simulink model "planner_contral"  (R2023b)
settings: Solver=FixedStepAuto  StartTime=0  StopTime=inf  FixedStep=0.001  RelTol=1e-3
undefined symbols (not defined in the file): aubr, c_factor, cf, cr, iniObsHeading1, iniObsHeading2, iniObsPos1, iniObsPos2, KD_PID_distance, KD_PID_speed, KI_PID_distance, KI_PID_speed, KP_PID_distance, KP_PID_speed, la, lb, LQR_K1, LQR_K2, LQR_K3, LQR_K4, m, rack_displacement, refInfo_obs1, refInfo_obs2, right_wheel_ground, rightWaypoints, tablebr, vubr, vx_break_point
libraries: Solver_SF x1
(part 2 of 8)

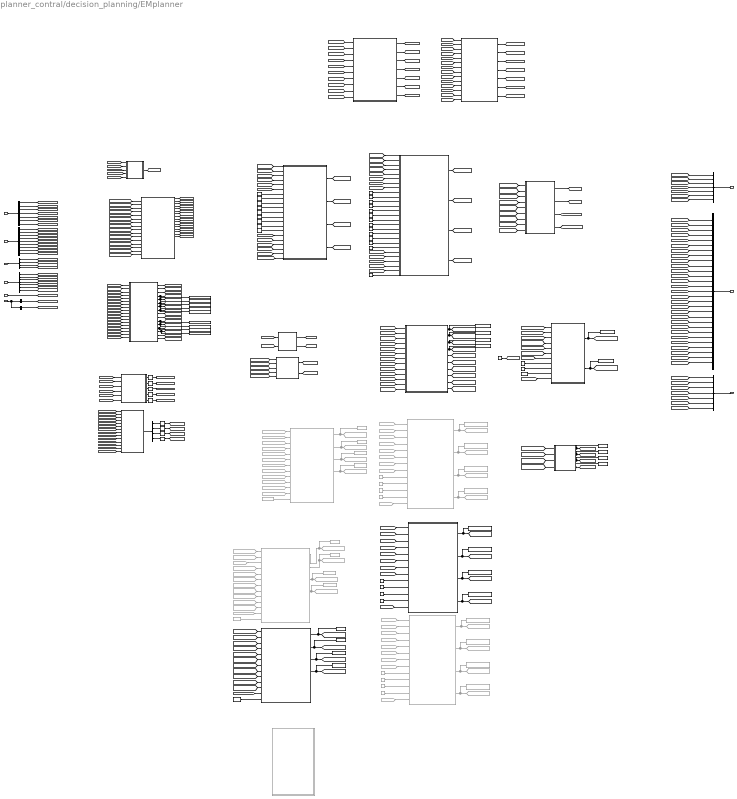
== system planner_contral/decision_planning/EMplanner ==
  note: 找到规划的起点
  note: 相对规划起点的时间序列
  note: 每个时刻对应的纵向位置
  note: 把QP的稀疏纵向轨迹增密、输出给后续控制器使用
  note: 在时域凸约束走廊内，对DP粗解进行平滑，求一条更连续、更舒适、更满足动力学约束的纵向轨迹。
  note: 路径速度拼接
  note: 在各个离散时刻上，静态/动态障碍物在ST图上占据的S下界和上界
  note: 输出
  note: 速度规划
  note: 路径索引到弧长的映射
  note: 当前规划起点处的纵向速度
  note: 当前规划起点横纵向位置
  note: 动态障碍物纵向速度
  note: 当前已生成的路径点，在 Frenet 下的轨迹
  note: 动态障碍物在 Frenet 下的位置和航向
  note: 静态障碍物在frenet下的位置和航向
  note: 把一条离散轨迹 (x,y) 转换成弧长坐标 s，并计算整条轨迹的总长度。
  note: 对给定的笛卡尔点，在参考线上搜索匹配点，并基于匹配点局部切线构造连续投影点，从而为后续 Frenet 坐标与动力学量转换提供基础几何信息。
  note: 点到参考线的匹配与投影函数
  note: 静态障碍物s
  note: 自车位置、航向角
  note: 上一周期轨迹 + 当前车辆状态
      | ↓
      | 判断是否还能沿用上一周期轨迹
      | ↓
      | 得到：
      | 1) 本周期规划起点
      | 2) 待拼接轨迹 stitch_trajectory
  note: 上一时刻规划的结果
      |
      | 当前时刻
      |
      | 自车信息
  note: 连续坐标：
      | s（沿道路方向）
      | l（横向偏移）
  note: origin = 自车在参考线上的投影点
  note: 这个模块的作用是：
      | 把参考线上的“点索引 i”转换成“弧长 s”，并且以自车投影点为 s=0
      | 构建以自车为原点的弧长坐标 s，实现“路径点编号 → 物理距离”的转换。。
  note: 输入
  note: 轨迹拼接计算模块
  note: accumulated_s计算模块
  note: 面向路径-速度解耦规划的障碍物预处理、参考线投影与动态轨迹构造模块
  note: 本周期规划起点
      |
      | 拼接轨迹
  note: （最多32）障碍物位置、速度、航向角
  note: 参考线位置、航向角、曲率
  note: 以自车为原点的弧长坐标 s
  note: 预测轨迹
  note: 静态障碍物l
  note: 静态障碍物航向角
  note: 动态障碍物s
  note: 动态障碍物l
  note: 动态障碍物s.
  note: 动态障碍物l.
  note: 动态障碍物航向角
  note: 本周期规划起点投影到参考线并转换到Frenet
  note: DP粗解决策+QP优化规划
      | 先离散决策，后连续优化。
  note: 每个时刻对应的纵向速度
  note: 每个时刻对应的纵向加速度
  note: 路径点的纵向坐标索引
  note: 当前规划时刻的绝对时间
  note: 把速度DP在ST图上的粗解转换成速度QP可直接使用的时域凸约束走廊。
  note: 路径规划
  referenceline_info : Inport
  location_info : Inport  Port=2
  perception info : Inport  Port=3
  pre_planning_info : Inport  Port=4
  current_time : Inport  Port=5
  visual_data : Inport  Port=6
  Bus Creator : BusCreator  Inputs=7
  Bus Creator1 : BusCreator  Inputs=29
  Bus Creator2 : BusCreator  Inputs=7
  Bus Selector : BusSelector  OutputSignals=smooth_ref_x,smooth_ref_y,smooth_ref_heading_,smooth_ref_kappa_,smooth_match_point_index,origin_x,origin_y
  Bus Selector1 : BusSelector  OutputSignals=ego_x,ego_y,ego_heading,ego_vx,ego_vy,ego_yaw_rate,ego_speed,ego_ax,ego_ay
  Bus Selector2 : BusSelector  OutputSignals=obs_x_set_gcs,obs_y_set_gcs,obs_velocity_set_gcs,obs_heading_set_gcs
  Bus Selector3 : BusSelector  OutputSignals=trajectory_x_gcs,trajectory_y_gcs,trajectory_heading_gcs,trajectory_kappa_gcs,trajectory_speed_gcs,trajectory_accel_gcs,trajectory_time_gcs
  Bus Selector4 : BusSelector  OutputSignals=preTraj_real1  OutputAsBus=on
  Bus Selector5 : BusSelector  OutputSignals=s_set,l_set,dl_set,ddl_set
  Bus Selector6 : BusSelector  OutputSignals=preTraj_real2  OutputAsBus=on
  Cartesian2Frenet : Subsystem
  Constant1 : Constant  Value=10
  Constant10 : Constant  Value=500
  Constant11 : Constant  Value=1000
  Constant12 : Constant  Value=500
  Constant13 : Constant  Value=100
  Constant{2,14,16,29} (4 alike) : Constant  Commented=on  Value=500
  Constant15 : Constant  Commented=on  Value=1000
  Constant17 : Constant  Commented=on  Value=100
  Constant18 : Constant  Commented=on  Value=0.2*9.8
  Constant28 : Constant  Commented=on  Value=1000
  Constant3 : Constant  Value=25
  Constant4 : Constant  Value=4000
  Constant5 : Constant  Value=100
  Constant6 : Constant  Value=1e8
  Constant60 : Constant  Value=1e8
  Constant61 : Constant  Value=1000
  Constant62 : Constant  Value=2
  Constant63 : Constant  Value=3
  Constant64 : Constant  Value=3
  Constant65 : Constant  Value=11
  Constant66 : Constant  Value=4
  Constant{67,76..78} (4 alike) : Constant  Value=15
  Constant68 : Constant  Value=1.2
  Constant69 : Constant  Value=0.1
  Constant7 : Constant  Commented=on  Value=0.2*9.8
  Constant70 : Constant  Value=0.02
  Constant71 : Constant  Value=2000
  Constant72 : Constant  Value=2500
  Constant73 : Constant  Value=50
  Constant74 : Constant  Value=20
  Constant75 : Constant  Value=5
  Constant79 : Constant  Value=2.5
  Constant8 : Constant  Value=0.2*9.8
  Constant80 : Constant  Value=2.5
  Constant81 : Constant  Value=1.6
  Constant9 : Constant  Commented=on  Value=100
  Frenet2Cartesian task : MATLAB Function  TreatAsAtomicUnit=on
  From{17,28,73,78} (4 alike) : From  Commented=on  GotoTag=obs_st_t_lb
  From{18,29,74,79} (4 alike) : From  Commented=on  GotoTag=obs_st_t_ub
  From{31,60,81,230} (4 alike) : From  Commented=on  GotoTag=dp_speed_s
  From231 : From  Commented=on  GotoTag=plan_start_s_dot
  From233 : From  Commented=on  GotoTag=plan_start_s_dot2
  From{32,63,82,234} (4 alike) : From  Commented=on  GotoTag=dp_speed_t
  From235 : From  Commented=on  GotoTag=s_lb
  From236 : From  Commented=on  GotoTag=s_ub
  From237 : From  Commented=on  GotoTag=s_dot_lb
  From238 : From  Commented=on  GotoTag=s_dot_ub
  From239 : From  Commented=on  GotoTag=reference_speed
  From25 : From  Commented=on  GotoTag=trajectory_kappa_init
  From26 : From  Commented=on  GotoTag=dynamic_s_lb
  From27 : From  Commented=on  GotoTag=dynaimc_s_ub
  From30 : From  Commented=on  GotoTag=path_s
  From33 : From  Commented=on  GotoTag=static_s_lb
  From34 : From  Commented=on  GotoTag=static_s_ub
  From61 : From  Commented=on  GotoTag=plan_start_s_dot
  From62 : From  Commented=on  GotoTag=plan_start_s_dot2
  From64 : From  Commented=on  GotoTag=s_lb
  From66 : From  Commented=on  GotoTag=s_ub
  From67 : From  Commented=on  GotoTag=s_dot_lb
  From71 : From  Commented=on  GotoTag=s_dot_ub
  From72 : From  Commented=on  GotoTag=reference_speed
  From75 : From  Commented=on  GotoTag=trajectory_kappa_init
  From76 : From  Commented=on  GotoTag=dynamic_s_lb
  From77 : From  Commented=on  GotoTag=dynaimc_s_ub
  From80 : From  Commented=on  GotoTag=path_s
  From83 : From  Commented=on  GotoTag=static_s_lb
  From84 : From  Commented=on  GotoTag=static_s_ub
  Goto146 : Goto  Commented=on  GotoTag=qp_s_init
  Goto147 : Goto  Commented=on  GotoTag=qp_s_dot_init
  Goto148 : Goto  Commented=on  GotoTag=qp_s_dot2_init
  Goto149 : Goto  Commented=on  GotoTag=relative_time_init
  Goto35 : Goto  Commented=on  GotoTag=s_lb
  Goto36 : Goto  Commented=on  GotoTag=s_ub
  Goto56 : Goto  Commented=on  GotoTag=s_dot_lb
  Goto57 : Goto  Commented=on  GotoTag=s_dot_ub
  Goto77 : Goto  Commented=on  GotoTag=qp_s_init
  Goto78 : Goto  Commented=on  GotoTag=qp_s_dot_init
  Goto79 : Goto  Commented=on  GotoTag=qp_s_dot2_init
  Goto80 : Goto  Commented=on  GotoTag=relative_time_init
  Goto81 : Goto  Commented=on  GotoTag=s_lb
  Goto82 : Goto  Commented=on  GotoTag=s_ub
  Goto83 : Goto  Commented=on  GotoTag=s_dot_lb
  Goto84 : Goto  Commented=on  GotoTag=s_dot_ub
  MATLAB Function1 : MATLAB Function  TreatAsAtomicUnit=on
  Selector{10..18} (9 alike) : Selector  InputPortWidth=128  IndexOptions=Index vector (dialog)  Indices=1  OutputSizes=1
  To Workspace : ToWorkspace  VariableName=log_dynamic_obs_s_set  SampleTime=-1
  To Workspace1 : ToWorkspace  VariableName=log_qp_s_init  SampleTime=-1
  To Workspace10 : ToWorkspace  VariableName=log_dp_speed_s  SampleTime=-1
  To Workspace11 : ToWorkspace  VariableName=log_dp_speed_t  SampleTime=-1
  To Workspace12 : ToWorkspace  Commented=on  VariableName=log_qp_s_init  SampleTime=-1
  To Workspace13 : ToWorkspace  Commented=on  VariableName=log_qp_s_dot_init  SampleTime=-1
  To Workspace14 : ToWorkspace  Commented=on  VariableName=log_qp_s_dot2_init  SampleTime=-1
  To Workspace15 : ToWorkspace  Commented=on  VariableName=log_relative_time_init  SampleTime=-1
  To Workspace16 : ToWorkspace  VariableName=log_s  SampleTime=-1
  To Workspace17 : ToWorkspace  VariableName=log_s_dot  SampleTime=-1
  To Workspace18 : ToWorkspace  VariableName=log_s_dot2  SampleTime=-1
  To Workspace19 : ToWorkspace  VariableName=log_relative_time  SampleTime=-1
  To Workspace2 : ToWorkspace  VariableName=log_static_s_lb  SampleTime=-1
  To Workspace20 : ToWorkspace  VariableName=log_dynamic_obs_l_set  SampleTime=-1
  To Workspace21 : ToWorkspace  VariableName=log_dynamic_obs_s_dot_set  SampleTime=-1
  To Workspace22 : ToWorkspace  VariableName=log_dynamic_obs_l_dot_set  SampleTime=-1
  To Workspace23 : ToWorkspace  VariableName=log_dynamic_obs_heading_set  SampleTime=-1
  To Workspace24 : ToWorkspace  VariableName=log_dynamic_obs_tra_x  SampleTime=-1
  To Workspace25 : ToWorkspace  VariableName=log_dynamic_obs_tra_y  SampleTime=-1
  To Workspace26 : ToWorkspace  VariableName=log_dynamic_obs_vx  SampleTime=-1
  To Workspace27 : ToWorkspace  VariableName=log_dynamic_obs_vy  SampleTime=-1
  To Workspace28 : ToWorkspace  Commented=on  VariableName=log_s_lb2  SampleTime=-1
  To Workspace29 : ToWorkspace  VariableName=log_s_lb  SampleTime=-1
  To Workspace3 : ToWorkspace  VariableName=log_static_s_ub  SampleTime=-1
  To Workspace30 : ToWorkspace  VariableName=log_s_ub  SampleTime=-1
  To Workspace31 : ToWorkspace  VariableName=log_s_dot_lb  SampleTime=-1
  To Workspace32 : ToWorkspace  VariableName=log_s_dot_ub  SampleTime=-1
  To Workspace33 : ToWorkspace  VariableName=log_qp_s_dot_init  SampleTime=-1
  To Workspace34 : ToWorkspace  VariableName=log_qp_s_dot2_init  SampleTime=-1
  To Workspace35 : ToWorkspace  VariableName=log_relative_time_init  SampleTime=-1
  To Workspace36 : ToWorkspace  Commented=on  VariableName=log_qp_s_init2  SampleTime=-1
  To Workspace37 : ToWorkspace  Commented=on  VariableName=log_qp_s_dot_init2  SampleTime=-1
  To Workspace38 : ToWorkspace  Commented=on  VariableName=log_qp_s_dot2_init2  SampleTime=-1
  To Workspace39 : ToWorkspace  Commented=on  VariableName=log_relative_time_init2  SampleTime=-1
  To Workspace4 : ToWorkspace  Commented=on  VariableName=log_s_lb  SampleTime=-1
  To Workspace40 : ToWorkspace  Commented=on  VariableName=log_s_ub2  SampleTime=-1
  To Workspace41 : ToWorkspace  Commented=on  VariableName=log_s_dot_lb2  SampleTime=-1
  To Workspace42 : ToWorkspace  Commented=on  VariableName=log_s_dot_ub2  SampleTime=-1
  To Workspace5 : ToWorkspace  Commented=on  VariableName=log_s_ub  SampleTime=-1
  To Workspace6 : ToWorkspace  Commented=on  VariableName=log_s_dot_lb  SampleTime=-1
  To Workspace7 : ToWorkspace  Commented=on  VariableName=log_s_dot_ub  SampleTime=-1
  To Workspace8 : ToWorkspace  VariableName=log_dynamic_s_lb  SampleTime=-1
  To Workspace9 : ToWorkspace  VariableName=log_dynamic_s_ub  SampleTime=-1
  calc path length and map between point and s : MATLAB Function  TreatAsAtomicUnit=on
  calc plan start info and stitch trajectory : MATLAB Function  TreatAsAtomicUnit=on
  calc speed planning start condition : MATLAB Function  TreatAsAtomicUnit=on
  generate convex space : MATLAB Function  Commented=on  TreatAsAtomicUnit=on
  generate convex space_base : MATLAB Function  TreatAsAtomicUnit=on
  generate convex space_new1 : MATLAB Function  Commented=on  TreatAsAtomicUnit=on
  generate st graph : MATLAB Function  TreatAsAtomicUnit=on
  generate st graph_base : MATLAB Function  Commented=on  TreatAsAtomicUnit=on
  genrate index to s : MATLAB Function  TreatAsAtomicUnit=on
  increase st point count : MATLAB Function  TreatAsAtomicUnit=on
  obs : Subsystem
  path and speed merge : MATLAB Function  TreatAsAtomicUnit=on
  path decision task : Subsystem
  path planning task : Subsystem
  spee planning with quadratic programming (qp) : MATLAB Function  Commented=on  TreatAsAtomicUnit=on
  spee planning with quadratic programming (qp)_1 : MATLAB Function  Commented=on  TreatAsAtomicUnit=on
  spee planning with quadratic programming (qp)_base : MATLAB Function  TreatAsAtomicUnit=on
  speed decision with dynamic planning(dp) : MATLAB Function  TreatAsAtomicUnit=on
  stitch trajectory : MATLAB Function  TreatAsAtomicUnit=on
  EM Planner result : Outport
  plot_visual : Outport  Port=2
  tra_ref_info : Outport  Port=3
  wires:
  referenceline_info/1 -> Bus Selector/1
  Bus Selector/1 -> [referenceline_x]  "<smooth_ref_x>"
  Bus Selector/2 -> [referenceline_y]  "<smooth_ref_y>"
  Bus Selector/3 -> [referenceline_heading]  "<smooth_ref_heading_>"
  Bus Selector/4 -> [referenceline_kappa]  "<smooth_ref_kappa_>"
  Bus Selector/5 -> [match_point_index]  "<smooth_match_point_index>"
  Bus Selector/6 -> [origin_x]  "<origin_x>"
  Bus Selector/7 -> [origin_y]  "<origin_y>"
  location_info/1 -> Bus Selector1/1
  Bus Selector1/1 -> [host_x]  "<ego_x>"
  Bus Selector1/2 -> [host_y]  "<ego_y>"
  Bus Selector1/3 -> [host_heading]  "<ego_heading>"
  Bus Selector1/4 -> [host_vx]  "<ego_vx>"
  Bus Selector1/5 -> [host_vy]  "<ego_vy>"
  Bus Selector1/6 -> [host_yawrate]  "<ego_yaw_rate>"
  Bus Selector1/7 -> [host_speed]  "<ego_speed>"
  Bus Selector1/8 -> [host_ax]  "<ego_ax>"
  Bus Selector1/9 -> [host_ay]  "<ego_ay>"
  pre_planning_info/1 -> Bus Selector3/1
  current_time/1 -> [current_time]
  [referenceline_y] -> genrate index to s/2(path_y)
  [referenceline_x] -> genrate index to s/1(path_x)
  genrate index to s/1(index2s) -> [index2s]
  [origin_y] -> genrate index to s/4(origin_y)
  [match_point_index] -> genrate index to s/5(origin_match_point_index)
  [origin_x] -> genrate index to s/3(origin_x)
  [host_ax] -> calc plan start info and stitch trajectory/14(host_ax)
  [host_ay] -> calc plan start info and stitch trajectory/15(host_ay)
  [pre_trajectory_x] -> calc plan start info and stitch trajectory/1(pre_trajectory_x)
  [pre_trajectory_y] -> calc plan start info and stitch trajectory/2(pre_trajectory_y)
  [pre_trajectory_heading] -> calc plan start info and stitch trajectory/3(pre_trajectory_heading)
  [pre_trajectory_kappa] -> calc plan start info and stitch trajectory/4(pre_trajectory_kappa)
  [pre_trajectory_speed] -> calc plan start info and stitch trajectory/5(pre_trajectory_velocity)
  [pre_trajectory_accel] -> calc plan start info and stitch trajectory/6(pre_trajectory_accel)
  [pre_trajectory_time] -> calc plan start info and stitch trajectory/7(pre_trajectory_time)
  [current_time] -> calc plan start info and stitch trajectory/8(current_time)
  [host_x] -> calc plan start info and stitch trajectory/9(host_x)
  [host_y] -> calc plan start info and stitch trajectory/10(host_y)
  [host_heading] -> calc plan start info and stitch trajectory/11(host_heading_xy)
  [host_vx] -> calc plan start info and stitch trajectory/12(host_vx)
  [host_vy] -> calc plan start info and stitch trajectory/13(host_vy)
  [host_speed] -> calc plan start info and stitch trajectory/16(host_speed)
  calc plan start info and stitch trajectory/1(plan_start_x) -> [plan_start_x_gcs]
  calc plan start info and stitch trajectory/2(plan_start_y) -> [plan_start_y_gcs]
  calc plan start info and stitch trajectory/4(plan_start_kappa) -> [plan_start_kappa_gcs]
  calc plan start info and stitch trajectory/5(plan_start_vx) -> [plan_start_vx_gcs]
  calc plan start info and stitch trajectory/6(plan_start_vy) -> [plan_start_vy_gcs]
  calc plan start info and stitch trajectory/7(plan_start_ax) -> [plan_start_ax_gcs]
  calc plan start info and stitch trajectory/8(plan_start_ay) -> [plan_start_ay_gcs]
  calc plan start info and stitch trajectory/9(plan_start_time) -> [plan_start_time]
  calc plan start info and stitch trajectory/11(stitch_y) -> [stitch_y_gcs]
  calc plan start info and stitch trajectory/12(stitch_heading) -> [stitch_heading_gcs]
  calc plan start info and stitch trajectory/13(stitch_kappa) -> [stitch_kappa_gcs]
  calc plan start info and stitch trajectory/14(stitch_speed) -> [stitch_speed_gcs]
  calc plan start info and stitch trajectory/15(stitch_accel) -> [stitch_accel_gcs]
  calc plan start info and stitch trajectory/16(stitch_time) -> [stitch_time]
  calc plan start info and stitch trajectory/3(plan_start_heading) -> [plan_start_heading_gcs]
  calc plan start info and stitch trajectory/10(stitch_x) -> [stitch_x_gcs]
  [plan_start_heading_gcs] -> calc speed planning start condition/5(plan_start_heading)
  [plan_start_ax_gcs] -> calc speed planning start condition/3(plan_start_ax)
  calc speed planning start condition/1(plan_start_s_dot) -> [plan_start_s_dot]
  [plan_start_vx_gcs] -> calc speed planning start condition/1(plan_start_vx)
  [plan_start_vy_gcs] -> calc speed planning start condition/2(plan_start_vy)
  [plan_start_ay_gcs] -> calc speed planning start condition/4(plan_start_ay)
  calc speed planning start condition/2(plan_start_s_dot2) -> [plan_start_s_dot2]
  calc path length and map between point and s/1(path_s_end) -> [path_s_end]
  calc path length and map between point and s/2(path_s) -> [path_s]  "path_s"
  [trajectory_x_init] -> calc path length and map between point and s/1(trajectory_x)
  [trajectory_y_init] -> calc path length and map between point and s/2(trajectory_y)
  Bus Creator/1 -> EM Planner result/1
  [trajectory_speed_final] -> Bus Creator/5  "trajectory_speed_gcs"
  [trajectory_time_final] -> Bus Creator/7  "trajectory_time_gcs"
  [trajectory_x_final] -> Bus Creator/1  "trajectory_x_gcs"
  [trajectory_kappa_final] -> Bus Creator/4  "trajectory_kappa_gcs"
  [trajectory_accel_final] -> Bus Creator/6  "trajectory_accel_gcs"
  [trajectory_heading_final] -> Bus Creator/3  "trajectory_heading_gcs"
  [trajectory_y_final] -> Bus Creator/2  "trajectory_y_gcs"
  Bus Selector3/1 -> [pre_trajectory_x]  "<trajectory_x_gcs>"
  Bus Selector3/7 -> [pre_trajectory_time]  "<trajectory_time_gcs>"
  Bus Selector3/6 -> [pre_trajectory_accel]  "<trajectory_accel_gcs>"
  Bus Selector3/5 -> [pre_trajectory_speed]  "<trajectory_speed_gcs>"
  Bus Selector3/4 -> [pre_trajectory_kappa]  "<trajectory_kappa_gcs>"
  Bus Selector3/3 -> [pre_trajectory_heading]  "<trajectory_heading_gcs>"
  Bus Selector3/2 -> [pre_trajectory_y]  "<trajectory_y_gcs>"
  [referenceline_x] -> obs/8(referenceline_x)
  [index2s] -> obs/12(index2s)
  [obs_velocity_set_gcs] -> obs/6(obs_velocity_set_gcs)
  [referenceline_heading] -> obs/10(referenceline_heading)
  [obs_heading_set_gcs] -> obs/7(obs_heading_set_gcs)
  [obs_x_set_gcs] -> obs/4(obs_x_set_gcs)
  [referenceline_kappa] -> obs/11(referenceline_kappa)
  [referenceline_y] -> obs/9(referenceline_y)
  obs/7(dynamic_obs_l_dot_set) -> [dynamic_obs_l_dot_set], To Workspace22/1
  [host_x] -> obs/1(host_x)
  obs/6(dynamic_obs_s_dot_set) -> [dynamic_obs_s_dot_set], To Workspace21/1
  obs/5(dynamic_obs_l_set) -> [dynamic_obs_l_set], To Workspace20/1
  [obs_y_set_gcs] -> obs/5(obs_y_set_gcs)
  obs/4(dynamic_obs_s_set) -> [dynamic_obs_s_set], To Workspace/1
  [host_heading] -> obs/3(host_heading_xy)
  [host_y] -> obs/2(host_y)
  Bus Selector2/4 -> [obs_heading_set_gcs]  "<obs_heading_set_gcs>"
  Bus Selector2/3 -> [obs_velocity_set_gcs]  "<obs_velocity_set_gcs>"
  Bus Selector2/1 -> [obs_x_set_gcs]  "<obs_x_set_gcs>"
  perception info/1 -> Bus Selector2/1
  Bus Selector2/2 -> [obs_y_set_gcs]  "<obs_y_set_gcs>"
  visual_data/1 -> Bus Selector6/1, Bus Selector4/1
  obs/1(static_obs_s_set) -> [static_obs_s_set]
  obs/2(static_obs_l_set) -> [static_obs_l_set]
  [path_s] -> obs/14(path_s)
  [preTraj1] -> obs/13(Pre_tra)
  [trajectory_x_init] -> obs/15(tra_x)
  [trajectory_y_init] -> obs/16(tra_y)
  [trajectory_kappa_init] -> obs/17(tra_kappa)
  [trajectory_heading_init] -> obs/18(tra_heaidng)
  obs/8(dynamic_obs_heading) -> [dynamic_obs_heading_set], To Workspace23/1
  obs/9(dynamic_obs_dl_set) -> [dynamic_obs_dl_set]
  obs/10(dynamic_obs_ddl_set) -> [dynamic_obs_ddl_set]
  obs/3(static_obs_heading_set) -> [static_obs_heading_set]
  obs/12(dynamic_obs_tra_y) -> [dynamic_obs_tra_y], To Workspace25/1
  obs/13(dynamic_obs_vx) -> To Workspace26/1, [dynamic_obs_vx]
  obs/14(dynamic_obs_vy) -> To Workspace27/1, [dynamic_obs_vy]
  obs/15(static_obs_x) -> [static_obs_x]
  obs/16(static_obs_y) -> [static_obs_y]
  obs/11(dynamic_obs_tra_x) -> [dynamic_obs_tra_x], To Workspace24/1
  [obs_st_t_ub] -> speed decision with dynamic planning(dp)/6(obs_st_t_ub)
  Constant6/1 -> speed decision with dynamic planning(dp)/10(w_cost_obs)
  [plan_start_s] -> generate st graph/12(plan_s)
  generate st graph/3(dynamic_obs_st_s_lb_set) -> To Workspace8/1, [dynamic_s_lb]
  generate st graph/7(static_obs_st_t_lb_set) -> [static_obs_st_t_in_set]
  [static_obs_l_set] -> generate st graph/2(static_obs_l)
  Constant5/1 -> speed decision with dynamic planning(dp)/9(w_cost_accel)
  speed decision with dynamic planning(dp)/2(dp_speed_t) -> To Workspace11/1, [dp_speed_t]
  generate st graph/2(static_obs_st_s_ub_set) -> To Workspace3/1, [static_s_ub]
  [obs_st_t_lb] -> speed decision with dynamic planning(dp)/5(obs_st_t_lb)
  [path_s] -> generate st graph/9(tra_path_indexs)
  generate st graph/1(static_obs_st_s_lb_set) -> To Workspace2/1, [static_s_lb]
  [qp_path_s_final] -> generate st graph/7(tra_s)
  Constant3/1 -> [reference_speed]
  [static_obs_s_set] -> generate st graph/1(static_obs_s)
  [plan_start_l] -> generate st graph/11(plan_l)
  [plan_start_s_dot] -> speed decision with dynamic planning(dp)/11(plan_start_s_dot)
  [dynaimc_s_ub] -> speed decision with dynamic planning(dp)/4(dynamic_obs_s_ub)
  speed decision with dynamic planning(dp)/1(dp_speed_s) -> To Workspace10/1, [dp_speed_s]
  [dynamic_s_lb] -> speed decision with dynamic planning(dp)/3(dynamic_obs_s_lb)
  [static_s_ub] -> speed decision with dynamic planning(dp)/2(static_obs_s_ub)
  Constant4/1 -> speed decision with dynamic planning(dp)/8(w_cost_ref_speed)
  [reference_speed] -> speed decision with dynamic planning(dp)/7(reference_speed_unlimit)
  [qp_path_l_final] -> generate st graph/8(tra_l)
  [static_obs_heading_set] -> generate st graph/3(static_obs_heading)
  [static_s_lb] -> speed decision with dynamic planning(dp)/1(static_obs_s_lb)
  [dynamic_obs_heading_set] -> generate st graph/6(dynamic_obs_heaidng_set)
  [dynamic_obs_l_set] -> generate st graph/5(dynamic_obs_l_set)
  [plan_start_s_dot] -> generate st graph/10(plan_s_dot)
  generate st graph/8(static_obs_st_t_ub_set) -> [static_obs_st_t_out_set]
  [dynamic_obs_s_dot_set] -> generate st graph/13(dynamic_obs_s_dot)
  generate st graph/4(dynamic_obs_st_s_ub_set) -> To Workspace9/1, [dynaimc_s_ub]
  [dynamic_obs_s_set] -> generate st graph/4(dynamic_obs_s_set)
  generate st graph/9(dynamic_obs_st_t_lb_set) -> [dynamic_obs_st_t_in_set]
  generate st graph/10(dynamic_obs_st_t_ub_set) -> [dynamic_obs_st_t_out_set]
  generate st graph/5(obs_st_t_lb_set) -> [obs_st_t_lb]
  generate st graph/6(obs_st_t_ub_set) -> [obs_st_t_ub]
  From236/1 -> spee planning with quadratic programming (qp)/6(s_ub)
  From230/1 -> spee planning with quadratic programming (qp)/3(dp_speed_s)
  From235/1 -> spee planning with quadratic programming (qp)/5(s_lb)
  From234/1 -> spee planning with quadratic programming (qp)/4(dp_speed_t)
  spee planning with quadratic programming (qp)/4(relative_time_init) -> To Workspace15/1, Goto149/1
  From239/1 -> spee planning with quadratic programming (qp)/13(speed_reference)
  From233/1 -> spee planning with quadratic programming (qp)/2(plan_start_s_dot2)
  From238/1 -> spee planning with quadratic programming (qp)/8(s_dot_ub)
  spee planning with quadratic programming (qp)/1(qp_s_init) -> To Workspace12/1, Goto146/1
  From237/1 -> spee planning with quadratic programming (qp)/7(s_dot_lb)
  From231/1 -> spee planning with quadratic programming (qp)/1(plan_start_s_dot)
  Constant9/1 -> spee planning with quadratic programming (qp)/9(w_cost_s_dot2)
  Constant29/1 -> spee planning with quadratic programming (qp)/11(w_cost_jerk)
  spee planning with quadratic programming (qp)/2(qp_s_dot_init) -> To Workspace13/1, Goto147/1
  spee planning with quadratic programming (qp)/3(qp_s_dot2_init) -> To Workspace14/1, Goto148/1
  Constant28/1 -> spee planning with quadratic programming (qp)/10(w_cost_v_ref)
  Constant2/1 -> spee planning with quadratic programming (qp)/12(w_ref_s)
  stitch trajectory/3(trajectory_heading_final) -> [trajectory_heading_final]
  [trajectory_x_init] -> path and speed merge/7(trajectory_x_init)
  [trajectory_kappa] -> stitch trajectory/4(trajectory_kappa)
  [trajectory_accel] -> stitch trajectory/6(trajectory_accel)
  [stitch_y_gcs] -> stitch trajectory/9(stitch_y)
  stitch trajectory/1(trajectory_x_final) -> [trajectory_x_final]
  stitch trajectory/2(trajectory_y_final) -> [trajectory_y_final]
  stitch trajectory/7(trajectory_time_final) -> [trajectory_time_final]
  [stitch_x_gcs] -> stitch trajectory/8(stitch_x)
  path and speed merge/4(trajectory_kappa) -> [trajectory_kappa]
  [trajectory_x] -> stitch trajectory/1(trajectory_x)
  stitch trajectory/4(trajectory_kappa_final) -> [trajectory_kappa_final]
  [relative_time] -> path and speed merge/4(relative_time)
  [s_dot2] -> path and speed merge/3(s_dot2)
  [plan_start_time] -> path and speed merge/5(current_time)
  increase st point count/3(s_dot2) -> To Workspace18/1, [s_dot2]
  [stitch_heading_gcs] -> stitch trajectory/10(stitch_heading)
  [trajectory_y] -> stitch trajectory/2(trajectory_y)
  increase st point count/2(s_dot) -> To Workspace17/1, [s_dot]
  [trajectory_y_init] -> path and speed merge/8(trajectory_y_init)
  stitch trajectory/5(trajectory_speed_final) -> [trajectory_speed_final]
  [trajectory_time] -> stitch trajectory/7(trajectory_time)
  [path_s] -> path and speed merge/6(path_s)
  [trajectory_heading_init] -> path and speed merge/9(trajectory_heading_init)
  path and speed merge/2(trajectory_y) -> [trajectory_y]
  [trajectory_heading] -> stitch trajectory/3(trajectory_heading)
  [stitch_kappa_gcs] -> stitch trajectory/11(stitch_kappa)
  path and speed merge/5(trajectory_speed) -> [trajectory_speed]
  path and speed merge/3(trajectory_heading) -> [trajectory_heading]
  [stitch_accel_gcs] -> stitch trajectory/13(stitch_accel)
  [stitch_speed_gcs] -> stitch trajectory/12(stitch_speed)
  [trajectory_speed] -> stitch trajectory/5(trajectory_speed)
  [s] -> path and speed merge/1(s)
  path and speed merge/7(trajectory_time) -> [trajectory_time]
  path and speed merge/6(trajectory_accel) -> [trajectory_accel]
  [qp_s_dot2_init] -> increase st point count/3(s_dot2_init)
  [relative_time_init] -> increase st point count/4(relative_time_init)
  [trajectory_kappa_init] -> path and speed merge/10(trajectory_kappa_init)
  [stitch_time] -> stitch trajectory/14(stitch_time)
  [qp_s_init] -> increase st point count/1(s_init)
  increase st point count/1(s) -> To Workspace16/1, [s]
  path and speed merge/1(trajectory_x) -> [trajectory_x]
  [s_dot] -> path and speed merge/2(s_dot)
  [qp_s_dot_init] -> increase st point count/2(s_dot_init)
  stitch trajectory/6(trajectory_accel_final) -> [trajectory_accel_final]
  increase st point count/4(relative_time) -> To Workspace19/1, [relative_time]
  [dynaimc_s_ub] -> Bus Creator1/17  "dynaimc_s_ub"
  [dynamic_s_lb] -> Bus Creator1/16  "dynamic_s_lb"
  [dp_path_s_final_ceshi] -> Bus Creator1/1  "dp_path_s_final_ceshi"
  [dp_path_l_final_ceshi] -> Bus Creator1/2  "dp_path_l_final_ceshi"
  [qp_path_s_final] -> Bus Creator1/3  "qp_path_s_final"
  [qp_path_l_final] -> Bus Creator1/4  "qp_path_l_final"
  [l_min] -> Bus Creator1/5  "l_min"
  [l_max] -> Bus Creator1/6  "l_max"
  [static_obs_s_set] -> Bus Creator1/7  "static_obs_s_set"
  [static_obs_l_set] -> Bus Creator1/8  "static_obs_l_set"
  [plan_start_s] -> Bus Creator1/9  "plan_start_s"
  [plan_start_l] -> Bus Creator1/10  "plan_start_l"
  [plan_start_dl] -> Bus Creator1/11  "plan_start_dl"
  [dynamic_obs_s_set] -> Bus Creator1/12  "dynamic_obs_s_set"
  [dynamic_obs_l_set] -> Bus Creator1/13  "dynamic_obs_l_set"
  [static_s_lb] -> Bus Creator1/14  "static_s_lb"
  [static_s_ub] -> Bus Creator1/15  "static_s_ub"
  [dp_speed_s] -> Bus Creator1/18  "dp_speed_s"
  [dp_speed_t] -> Bus Creator1/19  "dp_speed_t"
  [qp_s_init] -> Bus Creator1/20  "qp_s_init"
  [relative_time_init] -> Bus Creator1/21  "relative_time_init"
  [obs_st_t_lb] -> Bus Creator1/22  "obs_st_t_lb"
  [obs_st_t_ub] -> Bus Creator1/23  "obs_st_t_ub"
  [static_obs_st_t_in_set] -> Bus Creator1/24  "static_obs_st_t_in_set"
  [static_obs_st_t_out_set] -> Bus Creator1/25  "static_obs_st_t_out_set"
  [dynamic_obs_st_t_in_set] -> Bus Creator1/26  "dynamic_obs_st_t_in_set"
  [dynamic_obs_st_t_out_set] -> Bus Creator1/27  "dynamic_obs_st_t_out_set"
  [s_lb] -> Bus Creator1/28  "s_lb"
  [s_ub] -> Bus Creator1/29  "s_ub"
  Bus Creator1/1 -> plot_visual/1
  [referenceline_x] -> Bus Creator2/3  "referenceline_x"
  [trajectory_x_final] -> Bus Creator2/5  "trajectory_x_final"
  [host_y] -> Bus Creator2/2  "host_y"
  [referenceline_y] -> Bus Creator2/4  "referenceline_y"
  [trajectory_y_final] -> Bus Creator2/6  "trajectory_y_final"
  [host_x] -> Bus Creator2/1  "host_x"
  Bus Creator2/1 -> tra_ref_info/1
  [host_heading] -> Bus Creator2/7  "host_heading"
  path planning task/1(qp_path_s_final) -> [qp_path_s_final]
  Constant79/1 -> path planning task/17(host_d1)
  MATLAB Function1/4(proj_heading_set) -> Selector13/1
  [qp_path_s_final] -> Frenet2Cartesian task/1(s_set)
  [qp_path_dl_final] -> Frenet2Cartesian task/3(dl_set)
  [referenceline_heading] -> MATLAB Function1/5(frenet_path_heading)
  Frenet2Cartesian task/1(x_set) -> [trajectory_x_init]
  [referenceline_y] -> MATLAB Function1/4(frenet_path_y)
  [plan_start_match_point_index] -> Cartesian2Frenet/9(proj_match_point_index_set)
  [plan_start_vy_gcs] -> Cartesian2Frenet/4(vy_set)
  Selector11/1 -> [plan_start_proj_x]
  [referenceline_y] -> Cartesian2Frenet/8(frenet_path_y)
  [referenceline_x] -> Frenet2Cartesian task/5(frenet_path_x)
  [referenceline_kappa] -> Frenet2Cartesian task/8(frenet_path_kappa)
  Frenet2Cartesian task/2(y_set) -> [trajectory_y_init]
  MATLAB Function1/5(proj_kappa_set) -> Selector14/1
  [referenceline_x] -> Cartesian2Frenet/7(frenet_path_x)
  Bus Selector5/4 -> Selector18/1  "<ddl_set>"
  [plan_start_x_gcs] -> MATLAB Function1/1(x_set)
  Frenet2Cartesian task/4(kappa_set) -> [trajectory_kappa_init]
  [index2s] -> Frenet2Cartesian task/9(index2s)
  Bus Selector5/2 -> Selector16/1  "<l_set>"
  [plan_start_ax_gcs] -> Cartesian2Frenet/5(ax_set)
  [plan_start_vx_gcs] -> Cartesian2Frenet/3(vx_set)
  Selector15/1 -> [plan_start_s]
  Selector14/1 -> [plan_start_proj_kappa]
  Selector16/1 -> [plan_start_l]
  [plan_start_ay_gcs] -> Cartesian2Frenet/6(ay_set)
  [plan_start_proj_y] -> Cartesian2Frenet/11(proj_y_set)
  Selector17/1 -> [plan_start_dl]
  [index2s] -> Cartesian2Frenet/14(index2s)
  [referenceline_y] -> Frenet2Cartesian task/6(frenet_path_y)
  [dynamic_obs_s_dot_set] -> path decision task/18(dynamic_s_dot)
  MATLAB Function1/1(match_point_index_set) -> Selector10/1
  MATLAB Function1/2(proj_x_set) -> Selector11/1
  path decision task/1(dp_path_s_final) -> [dp_path_s_final_ceshi]
  [qp_path_ddl_final] -> Frenet2Cartesian task/4(ddl_set)
  Bus Selector5/1 -> Selector15/1  "<s_set>"
  [plan_start_s] -> path planning task/5(plan_start_s)
  Selector18/1 -> [plan_start_ddl]
  Constant64/1 -> path decision task/11(dp_cost_ref)
  [plan_start_s] -> path decision task/3(plan_start_s)
  Constant76/1 -> path planning task/14(qp_cost_endl)
  [referenceline_kappa] -> MATLAB Function1/6(frenet_path_kappa)
  Bus Selector5/3 -> Selector17/1  "<dl_set>"
  Constant74/1 -> path planning task/12(qp_cost_dddl)
  [plan_start_dl] -> path decision task/5(plan_start_dl)
  Constant66/1 -> path decision task/13(dp_col)
  [plan_start_proj_kappa] -> Cartesian2Frenet/13(proj_kappa_set)
  [dynamic_obs_l_dot_set] -> path decision task/19(dynamic_l_dot)
  Constant62/1 -> path decision task/9(dp_cost_ddl)
  path planning task/2(qp_path_l_final) -> [qp_path_l_final]
  path decision task/3(dp_path_dl_final) -> [dp_path_dl_final_ceshi]
  Constant81/1 -> path planning task/19(host_w)
  [dynamic_obs_s_set] -> path decision task/16(dynamic_s)
  Constant68/1 -> path decision task/15(dp_sample_l)
  [static_obs_s_set] -> path decision task/1(static_obs_s_set)
  Constant67/1 -> path decision task/14(dp_sample_s)
  path planning task/4(qp_path_ddl_final) -> [qp_path_ddl_final]
  [static_obs_l_set] -> path planning task/4(static_obs_l_set)
  [dynamic_obs_l_set] -> path decision task/17(dynamic_l)
  Constant71/1 -> path planning task/9(qp_cost_l)
  [static_obs_s_set] -> path planning task/3(static_obs_s_set)
  [dp_path_s_final_ceshi] -> path planning task/1(dp_path_s_final)
  Constant78/1 -> path planning task/16(qp_cost_end_ddl)
  Constant69/1 -> path planning task/20(delta_dl_max)
  [plan_start_ddl] -> path planning task/8(plan_start_ddl)
  path decision task/2(dp_path_l_final) -> [dp_path_l_final_ceshi]
  [referenceline_heading] -> Frenet2Cartesian task/7(frenet_path_heading)
  Constant73/1 -> path planning task/11(qp_cost_ddl)
  [plan_start_dl] -> path planning task/7(plan_start_dl)
  MATLAB Function1/3(proj_y_set) -> Selector12/1
  Cartesian2Frenet/1(Cartesian2FrenetOut) -> Bus Selector5/1
  [dynamic_obs_s_set] -> path planning task/22(dynamic_s)
  Constant70/1 -> path planning task/21(delta_ddl_max)
  [dynamic_obs_heading_set] -> path planning task/26(dynamic_heading)
  [dynamic_obs_l_set] -> path planning task/23(dynamic_l)
  Selector13/1 -> [plan_start_proj_heading]
  [dp_path_l_final_ceshi] -> path planning task/2(dp_path_l_final)
  Constant60/1 -> path decision task/7(dp_cost_collision)
  Constant63/1 -> path decision task/10(dp_cost_dddl)
  path planning task/3(qp_path_dl_final) -> [qp_path_dl_final]
  [qp_path_l_final] -> Frenet2Cartesian task/2(l_set)
  [static_obs_l_set] -> path decision task/2(static_obs_l_set)
  [referenceline_x] -> MATLAB Function1/3(frenet_path_x)
  [plan_start_l] -> path decision task/4(plan_start_l)
  Constant77/1 -> path planning task/15(qp_cost_end_dl)
  [dynamic_obs_l_dot_set] -> path planning task/25(dynamic_l_dot)
  Selector10/1 -> [plan_start_match_point_index]
  Selector12/1 -> [plan_start_proj_y]
  [dynamic_obs_s_dot_set] -> path planning task/24(dynamic_s_dot)
  [plan_start_ddl] -> path decision task/6(plan_start_ddl)
  Frenet2Cartesian task/3(heading_set) -> [trajectory_heading_init]
  [plan_start_l] -> path planning task/6(plan_start_l)
  [plan_start_proj_heading] -> Cartesian2Frenet/12(proj_heading_set)
  path decision task/4(dp_path_ddl_final) -> [dp_path_ddl_final_ceshi]
  [dynamic_obs_heading_set] -> path decision task/21(dynamic_obs_heading)
  [plan_start_proj_x] -> Cartesian2Frenet/10(proj_x_set)
  Constant72/1 -> path planning task/10(qp_cost_dl)
  [plan_start_x_gcs] -> Cartesian2Frenet/1(x_set)
  [plan_start_y_gcs] -> MATLAB Function1/2(y_set)
  Constant1/1 -> path planning task/27(w_ref_dp)
  [static_obs_heading_set] -> path decision task/20(static_obs_heading)
  Constant65/1 -> path decision task/12(dp_row)
  [plan_start_y_gcs] -> Cartesian2Frenet/2(y_set)
  Constant80/1 -> path planning task/18(host_d2)
  Constant75/1 -> path planning task/13(qp_cost_centre)
  Constant61/1 -> path decision task/8(dp_cost_dl)
  From33/1 -> generate convex space/4(static_obs_s_lb)
  From31/1 -> generate convex space/1(dp_speed_s)
  From27/1 -> generate convex space/9(dynamic_obs_s_ub)
  From26/1 -> generate convex space/8(dynamic_obs_s_lb)
  From29/1 -> generate convex space/11(dynamic_obs_t_ub)
  From28/1 -> generate convex space/10(dynamic_obs_t_lb)
  From32/1 -> generate convex space/2(dp_speed_t)
  From34/1 -> generate convex space/5(static_obs_s_ub)
  From17/1 -> generate convex space/6(static_obs_t_lb)
  From30/1 -> generate convex space/3(path_index2s)
  From18/1 -> generate convex space/7(static_obs_t_ub)
  generate convex space/1(s_lb) -> Goto35/1, To Workspace4/1
  From25/1 -> generate convex space/12(trajectory_kappa_init)
  Constant7/1 -> generate convex space/13(max_lateral_accel)
  generate convex space/2(s_ub) -> Goto36/1, To Workspace5/1
  generate convex space/4(s_dot_ub) -> Goto57/1, To Workspace7/1
  generate convex space/3(s_dot_lb) -> Goto56/1, To Workspace6/1
  Bus Selector4/1 -> [preTraj1]
  Bus Selector6/1 -> [preTraj2]
  Constant8/1 -> generate convex space_base/13(max_lateral_accel)
  [trajectory_kappa_init] -> generate convex space_base/12(trajectory_kappa_init)
  [obs_st_t_ub] -> generate convex space_base/7(static_obs_t_ub)
  [path_s] -> generate convex space_base/3(path_index2s)
  [obs_st_t_lb] -> generate convex space_base/6(static_obs_t_lb)
  [static_s_ub] -> generate convex space_base/5(static_obs_s_ub)
  [dp_speed_t] -> generate convex space_base/2(dp_speed_t)
  [obs_st_t_lb] -> generate convex space_base/10(dynaimc_obs_t_lb)
  [obs_st_t_ub] -> generate convex space_base/11(dynaimc_obs_t_ub)
  [dynamic_s_lb] -> generate convex space_base/8(dynamic_obs_s_lb)
  [dynaimc_s_ub] -> generate convex space_base/9(dynamic_obs_s_ub)
  [dp_speed_s] -> generate convex space_base/1(dp_speed_s)
  [static_s_lb] -> generate convex space_base/4(static_obs_s_lb)
  generate convex space_base/3(s_dot_lb) -> To Workspace31/1, [s_dot_lb]
  generate convex space_base/4(s_dot_ub) -> To Workspace32/1, [s_dot_ub]
  generate convex space_base/2(s_ub) -> To Workspace30/1, [s_ub]
  generate convex space_base/1(s_lb) -> To Workspace29/1, [s_lb]
  spee planning with quadratic programming (qp)_base/3(qp_s_dot2_init) -> [qp_s_dot2_init], To Workspace34/1
  spee planning with quadratic programming (qp)_base/2(qp_s_dot_init) -> [qp_s_dot_init], To Workspace33/1
  spee planning with quadratic programming (qp)_base/1(qp_s_init) -> [qp_s_init], To Workspace1/1
  spee planning with quadratic programming (qp)_base/4(relative_time_init) -> [relative_time_init], To Workspace35/1
  Constant10/1 -> spee planning with quadratic programming (qp)_base/12(w_ref_s)
  Constant11/1 -> spee planning with quadratic programming (qp)_base/10(w_cost_v_ref)
  Constant12/1 -> spee planning with quadratic programming (qp)_base/11(w_cost_jerk)
  Constant13/1 -> spee planning with quadratic programming (qp)_base/9(w_cost_s_dot2)
  [plan_start_s_dot] -> spee planning with quadratic programming (qp)_base/1(plan_start_s_dot)
  [s_dot_lb] -> spee planning with quadratic programming (qp)_base/7(s_dot_lb)
  [s_dot_ub] -> spee planning with quadratic programming (qp)_base/8(s_dot_ub)
  [plan_start_s_dot2] -> spee planning with quadratic programming (qp)_base/2(plan_start_s_dot2)
  [reference_speed] -> spee planning with quadratic programming (qp)_base/13(speed_reference)
  [dp_speed_t] -> spee planning with quadratic programming (qp)_base/4(dp_speed_t)
  [s_lb] -> spee planning with quadratic programming (qp)_base/5(s_lb)
  [dp_speed_s] -> spee planning with quadratic programming (qp)_base/3(dp_speed_s)
  [s_ub] -> spee planning with quadratic programming (qp)_base/6(s_ub)
  Constant14/1 -> spee planning with quadratic programming (qp)_1/12(w_ref_s)
  Constant15/1 -> spee planning with quadratic programming (qp)_1/10(w_cost_v_ref)
  spee planning with quadratic programming (qp)_1/3(qp_s_dot2_init) -> Goto79/1, To Workspace38/1
  spee planning with quadratic programming (qp)_1/2(qp_s_dot_init) -> Goto78/1, To Workspace37/1
  Constant16/1 -> spee planning with quadratic programming (qp)_1/11(w_cost_jerk)
  Constant17/1 -> spee planning with quadratic programming (qp)_1/9(w_cost_s_dot2)
  From61/1 -> spee planning with quadratic programming (qp)_1/1(plan_start_s_dot)
  From67/1 -> spee planning with quadratic programming (qp)_1/7(s_dot_lb)
  spee planning with quadratic programming (qp)_1/1(qp_s_init) -> Goto77/1, To Workspace36/1
  From71/1 -> spee planning with quadratic programming (qp)_1/8(s_dot_ub)
  From62/1 -> spee planning with quadratic programming (qp)_1/2(plan_start_s_dot2)
  From72/1 -> spee planning with quadratic programming (qp)_1/13(speed_reference)
  spee planning with quadratic programming (qp)_1/4(relative_time_init) -> Goto80/1, To Workspace39/1
  From63/1 -> spee planning with quadratic programming (qp)_1/4(dp_speed_t)
  From64/1 -> spee planning with quadratic programming (qp)_1/5(s_lb)
  From60/1 -> spee planning with quadratic programming (qp)_1/3(dp_speed_s)
  From66/1 -> spee planning with quadratic programming (qp)_1/6(s_ub)
  generate convex space_new1/1(s_lb) -> Goto81/1, To Workspace28/1
  generate convex space_new1/2(s_ub) -> Goto82/1, To Workspace40/1
  generate convex space_new1/4(s_dot_ub) -> Goto84/1, To Workspace42/1
  generate convex space_new1/3(s_dot_lb) -> Goto83/1, To Workspace41/1
  From83/1 -> generate convex space_new1/4(static_obs_s_lb)
  From81/1 -> generate convex space_new1/1(dp_speed_s)
  From77/1 -> generate convex space_new1/9(dynamic_obs_s_ub)
  From76/1 -> generate convex space_new1/8(dynamic_obs_s_lb)
  From79/1 -> generate convex space_new1/11(dynamic_obs_t_ub)
  From78/1 -> generate convex space_new1/10(dynamic_obs_t_lb)
  From82/1 -> generate convex space_new1/2(dp_speed_t)
  From84/1 -> generate convex space_new1/5(static_obs_s_ub)
  From73/1 -> generate convex space_new1/6(static_obs_t_lb)
  From80/1 -> generate convex space_new1/3(path_index2s)
  From74/1 -> generate convex space_new1/7(static_obs_t_ub)
  From75/1 -> generate convex space_new1/12(trajectory_kappa_init)
  Constant18/1 -> generate convex space_new1/13(max_lateral_accel)

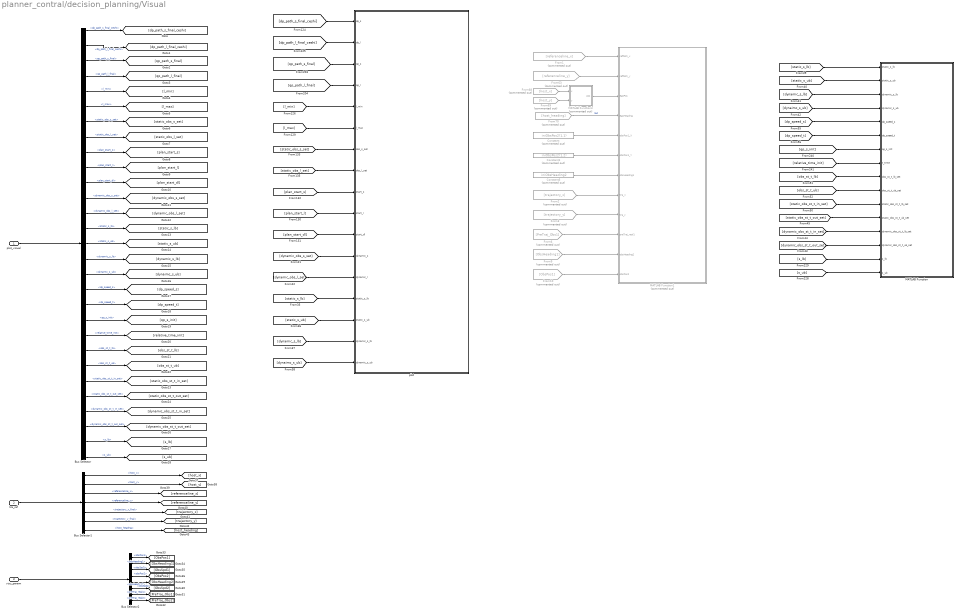
== system planner_contral/decision_planning/Visual ==
  plot_visual : Inport
  tra_ref : Inport  Port=2
  visu_param : Inport  Port=3
  Bus Selector : BusSelector  OutputSignals=dp_path_s_final_ceshi,dp_path_l_final_ceshi,qp_path_s_final,qp_path_l_final,l_min,l_max,static_obs_s_set,static_obs_l_set,plan_start_s,plan_start_l,plan_start_dl,dynamic_obs_s_set,dynamic_obs_l_set,static_s_lb,static_s_ub,dynamic_s_lb,dynaimc_s_ub,dp_speed_s,dp_speed_t,qp_s_init,relative_time_init,obs_st_t_lb,obs_st_t_ub,static_obs_st_t_in_set,static_obs_st_t_out_set,dynamic_obs_st_t_in_set,dynamic_obs_st_t_out_set,s_lb,s_ub
  Bus Selector1 : BusSelector  OutputSignals=host_x,host_y,referenceline_x,referenceline_y,trajectory_x_final,trajectory_y_final,host_heading
  Bus Selector2 : BusSelector  OutputSignals=obsPos1,obsHeading1,obsSpd1,obsPos2,obsHeading2,obsSpd2,preTraj_real1,preTraj_real2
  Constant : Constant  Commented=on  Value=iniObsPos2(1,1)
  Constant1 : Constant  Commented=on  Value=iniObsPos2(1,2)
  Constant5 : Constant  Commented=on  Value=iniObsHeading2
  From1 : From  Commented=on  GotoTag=referenceline_x
  From10 : From  Commented=on  GotoTag=ObsPos1
  From2 : From  Commented=on  GotoTag=trajectory_x
  From3 : From  Commented=on  GotoTag=trajectory_y
  From6 : From  Commented=on  GotoTag=PreTraj_Obs1
  From63 : From  Commented=on  GotoTag=referenceline_y
  From68 : From  Commented=on  GotoTag=host_x
  From69 : From  Commented=on  GotoTag=host_y
  From70 : From  Commented=on  GotoTag=host_heading
  From9 : From  Commented=on  GotoTag=ObsHeading1
  MATLAB Function : MATLAB Function  TreatAsAtomicUnit=on
  MATLAB Function1 : MATLAB Function  Commented=on  TreatAsAtomicUnit=on
  MATLAB Function3 : MATLAB Function  Commented=on  TreatAsAtomicUnit=on
  plot : MATLAB Function  TreatAsAtomicUnit=on
  wires:
  [qp_s_init] -> MATLAB Function/7(qp_s_init)
  [dp_speed_s] -> MATLAB Function/5(dp_speed_s)
  [dp_speed_t] -> MATLAB Function/6(dp_speed_t)
  [dynamic_obs_l_set] -> plot/13(dynamic_l)
  [qp_path_l_final] -> plot/4(qp_l)
  [s_ub] -> MATLAB Function/16(s_ub)
  [dp_path_l_final_ceshi] -> plot/2(dp_l)
  [static_obs_st_t_in_set] -> MATLAB Function/11(static_obs_st_t_lb_set)
  [static_s_ub] -> plot/15(static_s_ub)
  [dynaimc_s_ub] -> plot/17(dynamic_s_ub)
  [plan_start_s] -> plot/9(start_s)
  [obs_st_t_ub] -> MATLAB Function/10(obs_st_t_ub_set)
  [s_lb] -> MATLAB Function/15(s_lb)
  [qp_path_s_final] -> plot/3(qp_s)
  [dynamic_obs_st_t_in_set] -> MATLAB Function/13(dynamic_obs_st_t_lb_set)
  [relative_time_init] -> MATLAB Function/8(t_time)
  [obs_st_t_lb] -> MATLAB Function/9(obs_st_t_lb_set)
  [dynaimc_s_ub] -> MATLAB Function/4(dynamic_s_ub)
  [static_s_ub] -> MATLAB Function/2(static_s_ub)
  [static_s_lb] -> plot/14(static_s_lb)
  [l_min] -> plot/5(l_min)
  [l_max] -> plot/6(l_max)
  [static_obs_l_set] -> plot/8(obs_l_set)
  [static_s_lb] -> MATLAB Function/1(static_s_lb)
  [dynamic_s_lb] -> plot/16(dynamic_s_lb)
  [static_obs_st_t_out_set] -> MATLAB Function/12(static_obs_st_t_ub_set)
  [dp_path_s_final_ceshi] -> plot/1(dp_s)
  [plan_start_l] -> plot/10(start_l)
  [static_obs_s_set] -> plot/7(obs_s_set)
  [dynamic_s_lb] -> MATLAB Function/3(dynamic_s_lb)
  [plan_start_dl] -> plot/11(start_dl)
  [dynamic_obs_st_t_out_set] -> MATLAB Function/14(dynamic_obs_st_t_ub_set)
  plot_visual/1 -> Bus Selector/1
  Bus Selector/1 -> [dp_path_s_final_ceshi]  "<dp_path_s_final_ceshi>"
  Bus Selector/2 -> [dp_path_l_final_ceshi]  "<dp_path_l_final_ceshi>"
  Bus Selector/3 -> [qp_path_s_final]  "<qp_path_s_final>"
  Bus Selector/4 -> [qp_path_l_final]  "<qp_path_l_final>"
  Bus Selector/5 -> [l_min]  "<l_min>"
  Bus Selector/6 -> [l_max]  "<l_max>"
  Bus Selector/7 -> [static_obs_s_set]  "<static_obs_s_set>"
  Bus Selector/8 -> [static_obs_l_set]  "<static_obs_l_set>"
  Bus Selector/9 -> [plan_start_s]  "<plan_start_s>"
  Bus Selector/10 -> [plan_start_l]  "<plan_start_l>"
  Bus Selector/11 -> [plan_start_dl]  "<plan_start_dl>"
  Bus Selector/12 -> [dynamic_obs_s_set]  "<dynamic_obs_s_set>"
  Bus Selector/13 -> [dynamic_obs_l_set]  "<dynamic_obs_l_set>"
  Bus Selector/14 -> [static_s_lb]  "<static_s_lb>"
  Bus Selector/15 -> [static_s_ub]  "<static_s_ub>"
  Bus Selector/16 -> [dynamic_s_lb]  "<dynamic_s_lb>"
  Bus Selector/17 -> [dynaimc_s_ub]  "<dynaimc_s_ub>"
  Bus Selector/18 -> [dp_speed_s]  "<dp_speed_s>"
  Bus Selector/19 -> [dp_speed_t]  "<dp_speed_t>"
  Bus Selector/20 -> [qp_s_init]  "<qp_s_init>"
  Bus Selector/21 -> [relative_time_init]  "<relative_time_init>"
  Bus Selector/22 -> [obs_st_t_lb]  "<obs_st_t_lb>"
  Bus Selector/23 -> [obs_st_t_ub]  "<obs_st_t_ub>"
  Bus Selector/24 -> [static_obs_st_t_in_set]  "<static_obs_st_t_in_set>"
  Bus Selector/25 -> [static_obs_st_t_out_set]  "<static_obs_st_t_out_set>"
  Bus Selector/26 -> [dynamic_obs_st_t_in_set]  "<dynamic_obs_st_t_in_set>"
  Bus Selector/27 -> [dynamic_obs_st_t_out_set]  "<dynamic_obs_st_t_out_set>"
  Bus Selector/28 -> [s_lb]  "<s_lb>"
  Bus Selector/29 -> [s_ub]  "<s_ub>"
  Constant1/1 -> MATLAB Function1/6(obsPos1_Y)
  Constant/1 -> MATLAB Function1/5(obsPos1_X)
  From70/1 -> MATLAB Function1/4(egoHeading)  "rad"
  From9/1 -> MATLAB Function1/11(obsHeading2)
  MATLAB Function3/1(pos) -> MATLAB Function1/3(egoPos)
  From10/1 -> MATLAB Function1/12(obsPos2)
  From6/1 -> MATLAB Function1/10(preTraj_real1)
  From68/1 -> MATLAB Function3/1(x)
  From69/1 -> MATLAB Function3/2(y)
  From2/1 -> MATLAB Function1/8(tra_x)
  From63/1 -> MATLAB Function1/2(refPath_y)
  From3/1 -> MATLAB Function1/9(tra_y)
  From1/1 -> MATLAB Function1/1(refPath_x)
  Bus Selector2/7 -> [PreTraj_Obs1]  "<preTraj_real1>"
  Bus Selector2/4 -> [ObsPos2]  "<obsPos2>"
  Bus Selector2/8 -> [PreTraj_Obs2]  "<preTraj_real2>"
  Bus Selector2/5 -> [ObsHeading2]  "<obsHeading2>"
  Bus Selector2/6 -> [ObsSpd2]  "<obsSpd2>"
  Bus Selector2/3 -> [ObsSpd1]  "<obsSpd1>"
  Bus Selector2/1 -> [ObsPos1]  "<obsPos1>"
  Bus Selector2/2 -> [ObsHeading1]  "<obsHeading1>"
  visu_param/1 -> Bus Selector2/1
  tra_ref/1 -> Bus Selector1/1
  Bus Selector1/1 -> [host_x]  "<host_x>"
  Bus Selector1/2 -> [host_y]  "<host_y>"
  Bus Selector1/3 -> [referenceline_x]  "<referenceline_x>"
  Bus Selector1/4 -> [referenceline_y]  "<referenceline_y>"
  Bus Selector1/5 -> [trajectory_x]  "<trajectory_x_final>"
  Bus Selector1/6 -> [trajectory_y]  "<trajectory_y_final>"
  Bus Selector1/7 -> [host_heading]  "<host_heading>"
  Constant5/1 -> MATLAB Function1/7(obsHeading1)
  [dynamic_obs_s_set] -> plot/12(dynamic_s)
